simulink model "DeathOrGlory"  (R2017b)
settings: Solver=ode3  StartTime=0.0  StopTime=inf  FixedStep=0.0005  RelTol=1e-3
values from neighbouring files (symbols this model uses):
  fs = 1000    [Acquisizione_segnale_per_SVM_prova.m]    (also in training.m; warmup.m)
  interval = 192    [warmup.m]
  null_sum_finger = null_base_finger(:,1)+null_base_finger(:,2)    [matrix_h_hand_config.m]
  null_sum_thumb = null_base_thumb(:,1)+null_base_thumb(:,2)    [matrix_h_hand_config.m]
  num_act = 30    [KinematicData.m]
  pseudo_inv_h_finger = pinv(h_finger)    [matrix_h_hand_config.m]
  pseudo_inv_h_thumb = pinv(h_thumb)    [matrix_h_hand_config.m]
  pseudo_inv_h_wrist = pinv(h_wrist)    [matrix_h_hand_config.m]
  pseudo_inv_trasp_h_finger = pinv(transp(h_finger))    [matrix_h_hand_config.m]
  pseudo_inv_trasp_h_thumb = pinv(transp(h_thumb))    [matrix_h_hand_config.m]
  pseudo_inv_trasp_h_wrist = pinv(transp(h_wrist))    [matrix_h_hand_config.m]
  sM = mean(train(:,1:end-1))    [SVM_crossValidation.m]    (also in training.m; warmup.m = 0)
  sS = std(train(:,1:end-1))    [SVM_crossValidation.m]    (also in training.m; warmup.m = 0)
  Temg = 0.0005    [START_parametri_simulink.mat]    (also in matrix_h_hand_config.m)
  Ts = 0.05    [KinematicData.m]    (also in START_parametri_simulink.mat)
  w = 20    [Acquisizione_segnale_per_SVM_prova.m]    (also in warmup.m)
libraries: simulink x28, dspindex x15, dspfdesign x2, simulink_need_slupdate x2, dspmlti4 x1, dspstat3 x1, dspsrcs4 x1, simulink_extras x1
(part 1 of 2)
settings Model: Creator=UMBERTO  LastModifiedBy=Enrico
settings DataIOCC: LimitDataPoints=on  SaveFormat=Array
settings OptimizationCC: BlockReduction=off  BooleanDataType=off  LifeSpan=inf
settings DebuggingCC: SaveWithParameterizedLinksMsg=none  UnderspecifiedInitializationDetection=Classic  MergeDetectMultiDrivingBlocksExec=none  SignalResolutionControl=TryResolveAllWithWarning  SFUnexpectedBacktrackingDiag=warning  SFNoUnconditionalDefaultTransitionDiag=warning  SFExecutionAtInitializationDiag=none
settings HardwareCC: ProdBitPerPointer=32  ProdBitPerSizeT=32  ProdBitPerPtrDiffT=32  ProdLargestAtomicFloat=None  ProdIntDivRoundTo=Undefined  ProdEndianess=Unspecified  ProdWordSize=32  ProdHWDeviceType=32-bit Generic  TargetBitPerPointer=64  TargetBitPerSizeT=64  TargetBitPerPtrDiffT=64  TargetLongLongMode=on  TargetIntDivRoundTo=Zero  TargetEndianess=LittleEndian  TargetWordSize=64  TargetHWDeviceType=MATLAB Host  ProdEqTarget=off
settings ModelReferenceCC: UpdateModelReferenceTargets=Force  PropagateSignalLabelsOutOfModel=off
settings CodeAppCC: StateflowObjectComments=on
settings GRTTargetCC: TargetLangStandard=C89/C90 (ANSI)  GeneratePreprocessorConditionals=Disable all
settings ConfigComp: CovMetricSettings=dw  CovHtmlReporting=on  CovSaveCumulativeToWorkspaceVar=on  CovSaveSingleToWorkspaceVar=on  CovExternalEMLEnable=off  CovSFcnEnable=off

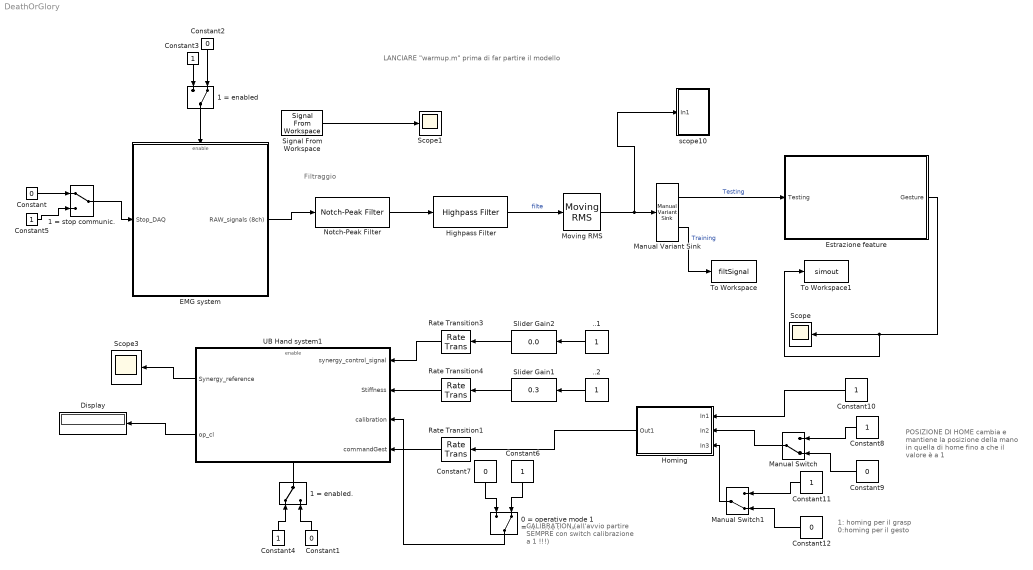
== system DeathOrGlory ==
  note: Filtraggio
  note: LANCIARE "warmup.m"
      | prima di far partire il modello
  note: CALIBRATION
      | (all'avvio partire SEMPRE con
      | switch calibrazione a 1 !!!)
  note: POSIZIONE DI HOME
      | cambia e mantiene la posizione della mano in quella di home fino a che il valore è a 1
  note: 1: homing per il grasp
      | 0:homing per il gesto
  ..1 : Constant  SampleTime=t
  ..2 : Constant  SampleTime=t
  0 = operative mode 1 = calibration mode : ManualSwitch  CurrentSetting=0
  1 = enabled : ManualSwitch  CurrentSetting=0  SampleTime=Temg
  1 = enabled. : ManualSwitch  SampleTime=t
  1 = stop communic. : ManualSwitch  SampleTime=Temg
  Constant : Constant  Value=0  SampleTime=Temg
  Constant1 : Constant  Value=0  SampleTime=t
  Constant{6,8,10..11} (4 alike) : Constant
  Constant12 : Constant  Value=0
  Constant2 : Constant  Value=0  SampleTime=Temg
  Constant3 : Constant  SampleTime=Temg
  Constant4 : Constant  SampleTime=t
  Constant5 : Constant  SampleTime=Temg
  Constant7 : Constant  Value=0
  Constant9 : Constant  Value=0
  Display : Display
  EMG system : Subsystem
  Estrazione feature : Subsystem
  Highpass Filter : dspfdesign/Highpass Filter  FilterType=FIR  DesignForMinimumOrder=on  FilterOrder=50  StopbandFrequency=w-5  PassbandFrequency=w  StopbandAttenuation=80  PassbandRipple=0.1  InheritSampleRate=off  SampleRate=fs  SimulateUsing=Interpreted execution  roundingMode=Floor  coeffsDataTypeStr=fixdt(1,16)
      settings: SourceProductName=DSP System Toolbox
  Homing : Subsystem
  Manual Variant Sink : simulink/Signal Routing/Manual Variant Sink  NumChoices=2  OverrideUsingVariant=V_1
      settings: SourceProductName=Simulink
  Manual Switch : ManualSwitch  CurrentSetting=0
  Manual Switch1 : ManualSwitch  CurrentSetting=0
  Moving RMS : dspstat3/Moving RMS  Method=Sliding window  SpecifyWindowLength=on  WindowLength=ws  ForgettingFactor=0.9  SimulateUsing=Code generation
      settings: SourceProductName=DSP System Toolbox  SourceProductBaseCode=DS
  Notch-Peak Filter : dspfdesign/Notch-Peak Filter  Specification=Quality factor and center frequency  Bandwidth=fs/2  QualityFactor=Q  CenterFrequency=notch  BandwidthCoefficient=0.72654  CenterFrequencyCoefficient=0  Output=Notch  InheritSampleRate=off  SampleRate=fs  SimulateUsing=Code generation
      settings: SourceProductName=DSP System Toolbox  SourceProductBaseCode=DS
  Rate Transition1 : RateTransition  OutPortSampleTime=Ts
  Rate Transition3 : RateTransition  OutPortSampleTime=Ts
  Rate Transition4 : RateTransition  OutPortSampleTime=Ts
  Scope : Scope
  Scope1 : Scope
  Scope3 : Scope
  Signal From Workspace : dspsrcs4/Signal From Workspace  X=cue_signal  Ts=1  nsamps=1  OutputAfterFinalValue=Cyclic repetition  ignoreOrWarnInputAndFrameLengths=off  OutputFrames=off
  Slider Gain1 : simulink/Math Operations/Slider Gain  gain=0.3  low=0  high=1
  Slider Gain2 : simulink/Math Operations/Slider Gain  gain=0.0  low=0  high=1
  To Workspace : ToWorkspace  VariableName=filtSignal  SampleTime=-1
      settings: Save2DSignal=2-D array (concatenate along first dimension)
  To Workspace1 : ToWorkspace  VariableName=simout  SampleTime=-1
      settings: Save2DSignal=2-D array (concatenate along first dimension)
  UB Hand system1 : Subsystem
  scope10 : Subsystem
  wires:
  Constant3/1 -> 1 = enabled/1
  Constant2/1 -> 1 = enabled/2
  1 = enabled/1 -> EMG system/Enable
  Constant5/1 -> 1 = stop communic./2
  Constant/1 -> 1 = stop communic./1
  1 = stop communic./1 -> EMG system/1(Stop_DAQ)
  Manual Variant Sink/2 -> To Workspace/1  "Training"
  Moving RMS/1 -> Manual Variant Sink/1, scope10/1(In1)
  Notch-Peak Filter/1 -> Highpass Filter/1
  Highpass Filter/1 -> Moving RMS/1  "filte"
  Constant4/1 -> 1 = enabled./1
  Slider Gain2/1 -> Rate Transition3/1
  ..1/1 -> Slider Gain2/1
  ..2/1 -> Slider Gain1/1
  Slider Gain1/1 -> Rate Transition4/1
  Constant6/1 -> 0 = operative mode 1 = calibration mode/2
  UB Hand system1/1(Synergy_reference) -> Scope3/1
  Constant1/1 -> 1 = enabled./2
  Rate Transition3/1 -> UB Hand system1/1(synergy_control_signal)
  Constant7/1 -> 0 = operative mode 1 = calibration mode/1
  Rate Transition4/1 -> UB Hand system1/2(Stiffness)
  UB Hand system1/2("op_cl ") -> Display/1
  0 = operative mode 1 = calibration mode/1 -> UB Hand system1/3(calibration)
  1 = enabled./1 -> UB Hand system1/Enable
  Rate Transition1/1 -> UB Hand system1/4(commandGest)
  Manual Variant Sink/1 -> Estrazione feature/1(Testing)  "Testing"
  Estrazione feature/1(Gesture) -> To Workspace1/1, Scope/1
  Constant8/1 -> Manual Switch/1
  Constant9/1 -> Manual Switch/2
  Manual Switch/1 -> Homing/2(In2)
  Manual Switch1/1 -> Homing/3(In3)
  Constant12/1 -> Manual Switch1/2
  Constant11/1 -> Manual Switch1/1
  Homing/1(Out1) -> Rate Transition1/1
  Constant10/1 -> Homing/1(In1)
  Signal From Workspace/1 -> Scope1/1
  EMG system/1(RAW_signals (8ch)) -> Notch-Peak Filter/1

== system DeathOrGlory/EMG system ==
  Stop_DAQ : Inport
  Enable : EnablePort
  MATLAB Function : MATLAB Function  TreatAsAtomicUnit=on
  Mux : Mux  Inputs=8
  RAW_signals (8ch) : Outport
  wires:
  Stop_DAQ/1 -> MATLAB Function/1(u)
  MATLAB Function/4(ch4) -> Mux/4
  MATLAB Function/3(ch3) -> Mux/3
  MATLAB Function/5(ch5) -> Mux/5
  MATLAB Function/6(ch6) -> Mux/6
  MATLAB Function/2(ch2) -> Mux/2
  MATLAB Function/1(ch1) -> Mux/1
  MATLAB Function/7(ch7) -> Mux/7
  MATLAB Function/8(ch8) -> Mux/8
  Mux/1 -> RAW_signals (8ch)/1

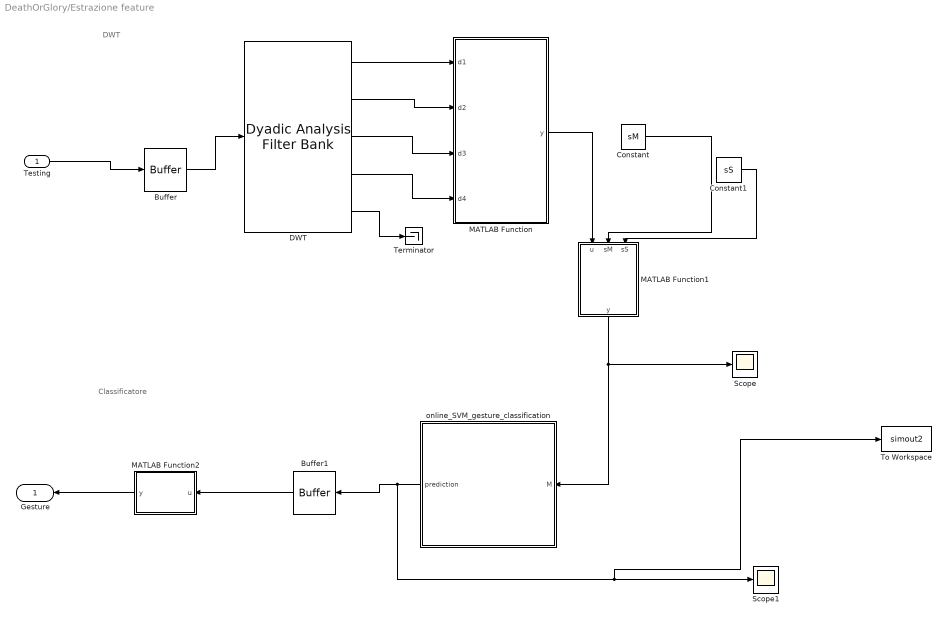
== system DeathOrGlory/Estrazione feature ==
  note: Classificatore
  note: DWT
  Testing : Inport
  Buffer : Buffer  N=interval  V=over  OutputFrames=off
  Buffer1 : Buffer  N=35  V=34
  Constant : Constant  Value=sM
  Constant1 : Constant  Value=sS
  DWT : dspmlti4/Dyadic Analysis Filter Bank  Wname=Daubechies  OrdRec_ordDec=[1 / 1]  Order=3  LPF="[0.0352   -0.0854   -0.1350   0.4599   0.8069   0.3327]"  HPF="[-0.3327    0.8069   -0.4599   -0.1350    0.0854    0.0352]"  NumLevels=level_dec  tree=Asymmetric  Output=Multiple ports  OutputFrames=off
      settings: SourceProductName=DSP System Toolbox  SourceProductBaseCode=DS
  MATLAB Function : MATLAB Function  TreatAsAtomicUnit=on
  MATLAB Function1 : MATLAB Function  TreatAsAtomicUnit=on
  MATLAB Function2 : MATLAB Function  TreatAsAtomicUnit=on
  Scope : Scope
  Scope1 : Scope
  Terminator : Terminator
  To Workspace : ToWorkspace  VariableName=simout2  SampleTime=-1
      settings: Save2DSignal=2-D array (concatenate along first dimension)
  online_SVM_gesture_classification : MATLAB Function  TreatAsAtomicUnit=on
  Gesture : Outport
  wires:
  DWT/5 -> Terminator/1
  DWT/3 -> MATLAB Function/3(d3)
  MATLAB Function/1(y) -> MATLAB Function1/1(u)
  DWT/1 -> MATLAB Function/1(d1)
  DWT/4 -> MATLAB Function/4(d4)
  DWT/2 -> MATLAB Function/2(d2)
  Buffer/1 -> DWT/1
  Testing/1 -> Buffer/1
  Buffer1/1 -> MATLAB Function2/1(u)
  online_SVM_gesture_classification/1(prediction) -> To Workspace/1, Scope1/1, Buffer1/1
  MATLAB Function1/1(y) -> Scope/1, online_SVM_gesture_classification/1(M)
  MATLAB Function2/1(y) -> Gesture/1
  Constant/1 -> MATLAB Function1/2(sM)
  Constant1/1 -> MATLAB Function1/3(sS)

== system DeathOrGlory/Homing ==
  In1 : Inport
  In2 : Inport  Port=2
  In3 : Inport  Port=3
  Constant : Constant  Value=8
  Constant1 : Constant
  Delay : Delay
  MATLAB Function : MATLAB Function  TreatAsAtomicUnit=on
  Scope : Scope
  Switch : Switch  Criteria=u2 ~= 0
  Switch1 : Switch  Criteria=u2 ~= 0
  Out1 : Outport
  wires:
  Delay/1 -> MATLAB Function/2(out)
  MATLAB Function/1(y) -> Switch/3
  In2/1 -> Switch/2
  Switch/1 -> Out1/1, Scope/1, Delay/1
  Constant1/1 -> Switch1/1
  Constant/1 -> Switch1/3
  In3/1 -> Switch1/2
  Switch1/1 -> Switch/1
  In1/1 -> MATLAB Function/1(u)

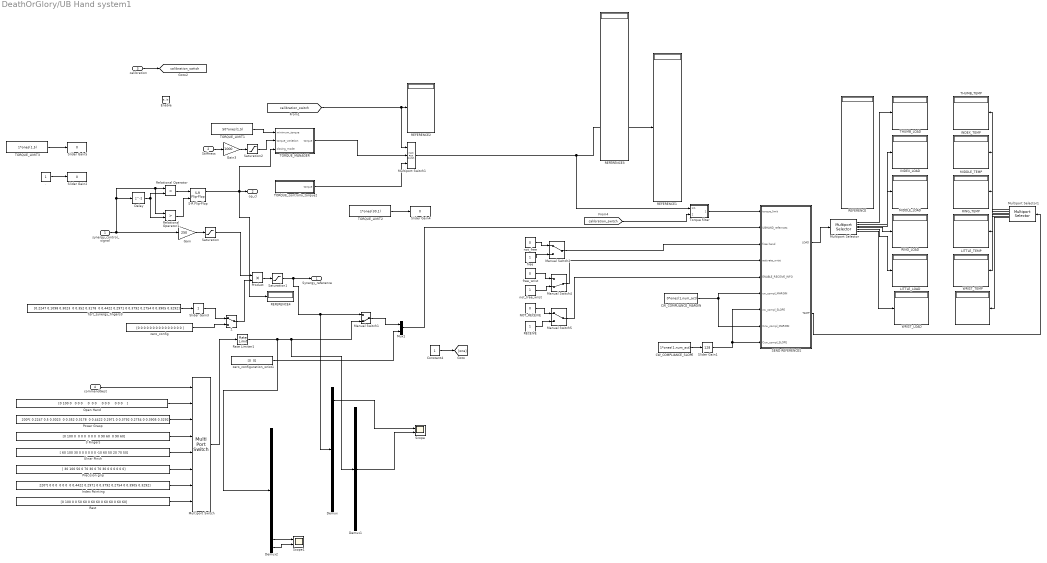
== system DeathOrGlory/UB Hand system1 ==
  synergy_control_signal : Inport
  Stiffness : Inport  Port=2
  calibration : Inport  Port=3
  commandGest : Inport  Port=4
  Enable : EnablePort
  . : Constant  SampleTime=t
  3 Fingers : Constant  Value="[0 100 0  0 0 0  0 0 0  0 90 60  0 90 60]"  SampleTime=t
  :1 : ManualSwitch  SampleTime=t
  CW_COMPLIANCE_MARGIN : Constant  Value=0*ones(1,num_act)
  CW_COMPLIANCE_SLOPE : Constant  Value=1*ones(1,num_act)
  Constant4 : Constant  SampleTime=t
  Delay : Delay  DelayLength=1  InitialCondition=0
  Demux : Demux  Outputs=15
  Demux1 : Demux  Outputs=15
  Demux2 : Demux  Outputs=15
  Gain : Gain  Gain=250
  Gain3 : Gain  Gain=1000
  INDEX_LOAD : Display
  INDEX_TEMP : Display
  Index Pointing : Constant  Value="220*[ 0 0 0  0 0 0  0 0.4422 0.2971 0 0.3792 0.2754 0 0.3905 0.3292]"  SampleTime=t
  LITTLE_LOAD : Display
  LITTLE_TEMP : Display
  MIDDLE_LOAD : Display
  MIDDLE_TEMP : Display
  Manual Switch1 : ManualSwitch  CurrentSetting=0
  Manual Switch2 : ManualSwitch  Description=SEND  SampleTime=t
      settings: AttributesFormatString=SEND
  Manual Switch4 : ManualSwitch  Description=SEND  CurrentSetting=0  SampleTime=t
      settings: AttributesFormatString=SEND
  Manual Switch5 : ManualSwitch  Description=SEND  SampleTime=t
      settings: AttributesFormatString=SEND
  Multiport Selector : dspindex/Multiport Selector  rowsOrCols=Rows  idxCellArray={ [1:5],[6:10],[11:15],[16:20],[21:25],[26:29]}  idxErrMode=Clip Index
  Multiport Selector1 : dspindex/Multiport Selector  rowsOrCols=Rows  idxCellArray={ [1:5],[6:10],[11:15],[16:20],[21:25],[26:29]}  idxErrMode=Clip Index
  Multiport Switch : MultiPortSwitch  DataPortOrder=Specify indices  Inputs=6  DataPortIndices={1,2,3,4,5,6,8}
  Multiport Switch1 : MultiPortSwitch  DataPortOrder=Zero-based contiguous  Inputs=2  DiagnosticForDefault=None
  Mux1 : Mux  Inputs=2
  NOT_RECEIVE : Constant  Value=0  SampleTime=t
  Open Hand : Constant  Value="[0 100 0   0 0 0     0  0 0     0 0 0     0 0 0    ]"  SampleTime=t
  Power Grasp : Constant  Value="200*[ 0.2247 0.5 0.3023  0 0.352 0.3178  0 0.4422 0.2971 0 0.3792 0.2754 0 0.3905 0.3292]"  SampleTime=t
  Precision grip : Constant  Value=[ 30 100 50 0 70 30 0 70 30 0 0 0 0 0 0]  SampleTime=t
  Product : Product  SampleTime=t
  RECEIVE : Constant  SampleTime=t
  REFERENCE{,1..4} (5 alike) : Display
  RING_LOAD : Display
  RING_TEMP : Display
  Rate Limiter1 : RateLimiter  RisingSlewLimit=80  FallingSlewLimit=-80  SampleTimeMode=inherited
  Relational Operator : RelationalOperator  Operator=<  OutDataTypeStr=boolean  RndMeth=Nearest
  Relational Operator1 : RelationalOperator  Operator=>  OutDataTypeStr=boolean  RndMeth=Nearest
  Rest : Constant  Value=[0 100 0 0 50 60 0 60 60 0 60 60 0 60 60]  SampleTime=t
  S-R Flip-Flop : simulink_extras/Flip Flops/S-R Flip-Flop  initial_condition=0
  SEND REFERENCES : Subsystem
  Saturation : Saturate  UpperLimit=250  LowerLimit=0
  Saturation1 : Saturate  UpperLimit=250  LowerLimit=0
  Saturation2 : Saturate  UpperLimit=1000  LowerLimit=0
  Scope : Scope  NumInputPorts=2
  Scope1 : Scope  NumInputPorts=2
  Slider Gain1 : simulink/Math Operations/Slider Gain  gain=128  low=0  high=128
  Slider Gain2 : simulink/Math Operations/Slider Gain  gain=0  low=0  high=1000
  Slider Gain3 : simulink/Math Operations/Slider Gain  gain=1  low=0  high=250
  Slider Gain4 : simulink/Math Operations/Slider Gain  gain=0  low=0  high=1000
  Slider Gain5 : simulink/Math Operations/Slider Gain  gain=0  low=0  high=1000
  THUMB_LOAD : Display
  THUMB_TEMP : Display
  TORQUE_LIMIT1 : Constant  Value=50*ones(1,5)  SampleTime=t
  TORQUE_LIMIT2 : Constant  Value=1*ones(30,1)  SampleTime=t
  TORQUE_LIMIT3 : Constant  Value=1*ones(1,5)  SampleTime=t
  TORQUE_MANAGER : Subsystem
  TORQUE_controllo_torque2 : Subsystem
  Torque filter : Subsystem
  Ulnar Pinch : Constant  Value=[ 60 100 30 0 0 0 0 0 0 -10 60 50 20 70 50]  SampleTime=t
  WRIST_LOAD : Display
  WRIST_TEMP : Display
  fisrt_synergy_fingers3 : Constant  Value="[0.2247 0.1098 0.3023  0 0.352 0.3178  0 0.4422 0.2971 0 0.3792 0.2754 0 0.3905 0.3292]'"  SampleTime=t
  free : Constant  SampleTime=t
  free_wrist : Constant  Value=0  SampleTime=t
  not_free : Constant  Value=0  SampleTime=t
  not_free_wrist : Constant  SampleTime=t
  zero_config : Constant  Value="[0 0 0   0 0 0     0  0 0     0 0 0     0 0 0    ]"  SampleTime=t
  zero_configuration_wrist1 : Constant  Value="[0  0]"  SampleTime=t
  Synergy_reference : Outport
  "op_cl " : Outport  Port=2
  tag scope: calibration_switch=global
  wires:
  Constant4/1 -> [one]
  not_free/1 -> Manual Switch2/1
  free/1 -> Manual Switch2/2
  Manual Switch2/1 -> SEND REFERENCES/3(free hand)
  free_wrist/1 -> Manual Switch4/1
  Manual Switch4/1 -> SEND REFERENCES/4(activate_wrist)
  NOT_RECEIVE/1 -> Manual Switch5/1
  RECEIVE/1 -> Manual Switch5/2
  Manual Switch5/1 -> SEND REFERENCES/5(ENABLE_RECEIVE_INFO)
  not_free_wrist/1 -> Manual Switch4/2
  zero_configuration_wrist1/1 -> Mux1/2
  Gain/1 -> Saturation/1
  SEND REFERENCES/2(TEMP) -> Multiport Selector1/1
  Multiport Selector/1 -> THUMB_LOAD/1
  Multiport Selector/2 -> INDEX_LOAD/1
  Multiport Selector/3 -> MIDDLE_LOAD/1
  Multiport Selector/4 -> RING_LOAD/1
  Multiport Selector/5 -> LITTLE_LOAD/1
  Multiport Selector/6 -> WRIST_LOAD/1
  Multiport Selector1/1 -> THUMB_TEMP/1
  Multiport Selector1/2 -> INDEX_TEMP/1
  Multiport Selector1/3 -> MIDDLE_TEMP/1
  Multiport Selector1/4 -> RING_TEMP/1
  Multiport Selector1/5 -> LITTLE_TEMP/1
  Multiport Selector1/6 -> WRIST_TEMP/1
  SEND REFERENCES/1(LOAD) -> Multiport Selector/1
  Saturation/1 -> Product/1
  CW_COMPLIANCE_SLOPE/1 -> Slider Gain1/1
  TORQUE_LIMIT1/1 -> TORQUE_MANAGER/1(minimum_torque)
  [calibration_switch] -> Multiport Switch1/1, REFERENCE2/1
  Product/1 -> Saturation1/1
  Saturation1/1 -> Demux/1, Manual Switch1/1, Synergy_reference/1
  TORQUE_controllo_torque2/1(torque) -> Multiport Switch1/3
  zero_config/1 -> :1/2
  :1/1 -> Product/2
  fisrt_synergy_fingers3/1 -> Slider Gain3/1
  TORQUE_LIMIT2/1 -> Slider Gain4/1
  TORQUE_LIMIT3/1 -> Slider Gain5/1
  ./1 -> Slider Gain2/1
  Saturation2/1 -> TORQUE_MANAGER/2(torque_variation)
  Mux1/1 -> SEND REFERENCES/2(UBHAND_refernces)
  CW_COMPLIANCE_MARGIN/1 -> SEND REFERENCES/6(cw_compl_MARGIN), SEND REFERENCES/8(Ccw_compl_MARGIN)
  Slider Gain1/1 -> SEND REFERENCES/7("cw_compl_SLOPE "), SEND REFERENCES/9(Ccw_compl_SLOPE)
  Torque filter/1(Out1) -> SEND REFERENCES/1(torque_limit)
  [calibration_switch] -> Torque filter/2("reset ")
  calibration/1 -> [calibration_switch]
  Multiport Switch1/1 -> Torque filter/1(In1), REFERENCE1/1
  TORQUE_MANAGER/1(torque) -> Multiport Switch1/2
  Gain3/1 -> Saturation2/1
  Stiffness/1 -> Gain3/1
  Slider Gain3/1 -> :1/1
  Delay/1 -> Relational Operator1/2, Relational Operator/2
  S-R Flip-Flop/1 -> TORQUE_MANAGER/3(closing_mode), "op_cl "/1, REFERENCE4/1
  Relational Operator/1 -> S-R Flip-Flop/1
  synergy_control_signal/1 -> Relational Operator1/1, Relational Operator/1, Delay/1, Gain/1
  Relational Operator1/1 -> S-R Flip-Flop/2
  Multiport Switch/1 -> Rate Limiter1/1
  Manual Switch1/1 -> Mux1/1
  Demux/2 -> Scope/1
  Demux1/8 -> Scope/2
  Open Hand/1 -> Multiport Switch/2
  Power Grasp/1 -> Multiport Switch/3
  3 Fingers/1 -> Multiport Switch/4
  Ulnar Pinch/1 -> Multiport Switch/5
  Precision grip/1 -> Multiport Switch/6
  Index Pointing/1 -> Multiport Switch/7
  Rest/1 -> Multiport Switch/8
  commandGest/1 -> Multiport Switch/1
  Rate Limiter1/1 -> Demux2/1, Demux1/1, Manual Switch1/2
  Demux2/14 -> Scope1/1
  Demux2/15 -> Scope1/2

== system DeathOrGlory/scope10 ==
  In1 : Inport
  Demux : Demux  Outputs=8
  Scope : Scope  NumInputPorts=8
  wires:
  In1/1 -> Demux/1
  Demux/7 -> Scope/7
  Demux/4 -> Scope/4
  Demux/5 -> Scope/5
  Demux/8 -> Scope/8
  Demux/1 -> Scope/1
  Demux/2 -> Scope/2
  Demux/6 -> Scope/6
  Demux/3 -> Scope/3

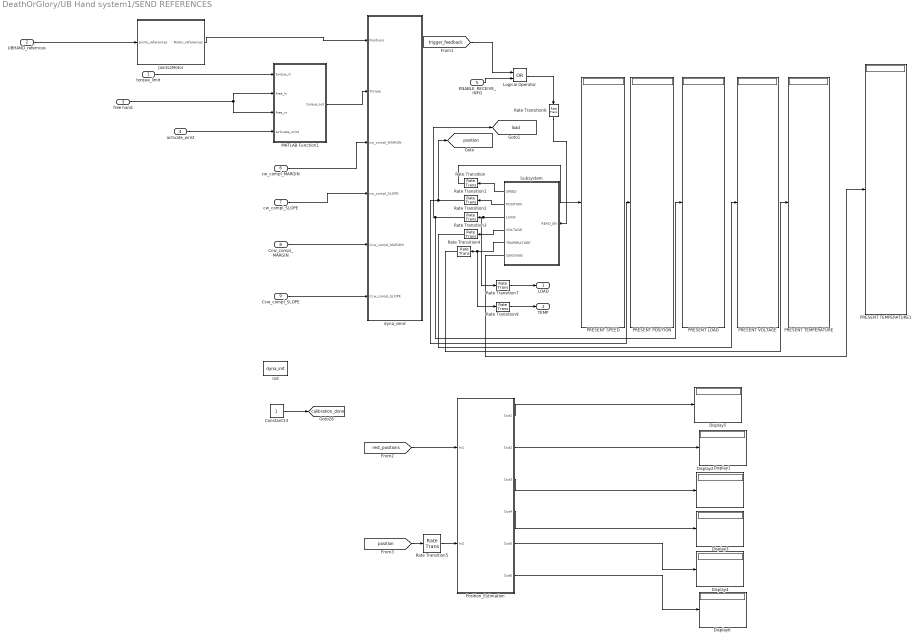
== system DeathOrGlory/UB Hand system1/SEND REFERENCES ==
  torque_limit : Inport
  UBHAND_refernces : Inport  Port=2
  free hand : Inport  Port=3
  activate_wrist : Inport  Port=4
  ENABLE_RECEIVE_INFO : Inport  Port=5
  cw_compl_MARGIN : Inport  Port=6
  "cw_compl_SLOPE " : Inport  Port=7
  Ccw_compl_MARGIN : Inport  Port=8
  Ccw_compl_SLOPE : Inport  Port=9
  Constant33 : Constant  SampleTime=Ts
  Display{1..6} (6 alike) : Display
  Init : M-S-Function  FunctionName=dyna_init  Parameters=5 1
  Joints2Motor : Subsystem
  Logical Operator : Logic  Operator=OR  AllPortsSameDT=off  OutDataTypeStr=boolean
  MATLAB Function1 : MATLAB Function  TreatAsAtomicUnit=on
  PRESENT LOAD : Display
  PRESENT POSITION : Display
  PRESENT SPEED : Display
  PRESENT TEMPERATURE : Display
  PRESENT TEMPERATURE1 : Display
  PRESENT VOLTAGE : Display
  Position_Estimation : Subsystem
  Rate Transition{,1..4,6..7,9} (8 alike) : RateTransition
  Rate Transition5 : RateTransition  OutPortSampleTime=Ts
  Subsystem : Subsystem  SystemSampleTime=0.1
  dyna_send : Subsystem
  LOAD : Outport
  TEMP : Outport  Port=2
  tag scope: calibration_done=global, load=global, position=global
  wires:
  torque_limit/1 -> MATLAB Function1/1(torque_in)
  Joints2Motor/1(Motor_references) -> dyna_send/1(Positions)
  ENABLE_RECEIVE_INFO/1 -> Logical Operator/2
  Logical Operator/1 -> Rate Transition6/1
  [trigger_feedback] -> Logical Operator/1
  activate_wrist/1 -> MATLAB Function1/4(activate_wrist)
  MATLAB Function1/1(torque_out) -> dyna_send/2(Torque)
  UBHAND_refernces/1 -> Joints2Motor/1(Joints_references)
  free hand/1 -> MATLAB Function1/3(free_rx), MATLAB Function1/2(free_lx)
  Constant33/1 -> [calibration_done]
  Subsystem/1(SPEED) -> Rate Transition/1
  Subsystem/2(POSITION) -> Rate Transition1/1
  Subsystem/3(LOAD) -> Rate Transition7/1, Rate Transition2/1
  Subsystem/4(VOLTAGE) -> Rate Transition3/1
  Subsystem/5(TEMPERATURE) -> Rate Transition4/1, Rate Transition9/1
  cw_compl_MARGIN/1 -> dyna_send/3(cw_compl_MARGIN)
  "cw_compl_SLOPE "/1 -> dyna_send/4(cw_compl_SLOPE)
  Ccw_compl_MARGIN/1 -> dyna_send/5(Ccw_compl_MARGIN)
  Ccw_compl_SLOPE/1 -> dyna_send/6(Ccw_compl_SLOPE)
  Position_Estimation/1(Out1) -> Display5/1
  Position_Estimation/2(Out2) -> Display1/1
  Position_Estimation/3(Out3) -> Display2/1
  Position_Estimation/4(Out4) -> Display3/1
  Position_Estimation/5(Out5) -> Display4/1
  Position_Estimation/6(Out6) -> Display6/1
  [rest_positions] -> Position_Estimation/1(In1)
  [position] -> Rate Transition5/1
  Rate Transition/1 -> PRESENT SPEED/1
  Rate Transition1/1 -> [position], PRESENT POSITION/1
  Rate Transition3/1 -> PRESENT VOLTAGE/1
  Rate Transition4/1 -> PRESENT TEMPERATURE/1
  Rate Transition5/1 -> Position_Estimation/2(In2)
  Rate Transition6/1 -> Subsystem/1(READ_EN)
  Rate Transition9/1 -> TEMP/1
  Rate Transition7/1 -> LOAD/1
  Rate Transition2/1 -> [load], PRESENT LOAD/1
  Subsystem/6(ISMOVING) -> PRESENT TEMPERATURE1/1

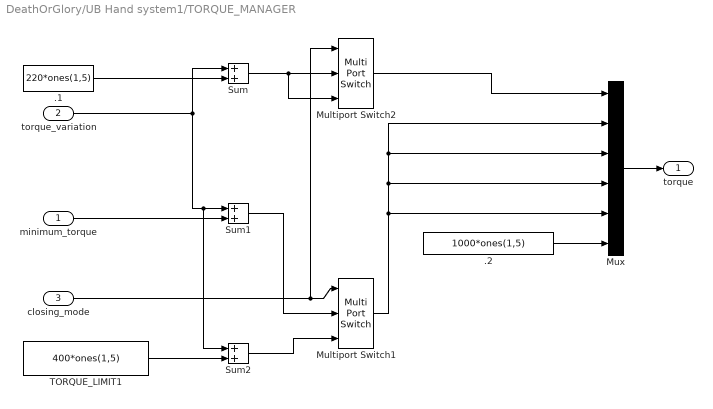
== system DeathOrGlory/UB Hand system1/TORQUE_MANAGER ==
  minimum_torque : Inport
  torque_variation : Inport  Port=2
  closing_mode : Inport  Port=3
  .1 : Constant  Value=220*ones(1,5)  SampleTime=t
  .2 : Constant  Value=1000*ones(1,5)  SampleTime=t
  Multiport Switch1 : MultiPortSwitch  DataPortOrder=Zero-based contiguous  Inputs=2  DiagnosticForDefault=None
  Multiport Switch2 : MultiPortSwitch  DataPortOrder=Zero-based contiguous  Inputs=2  DiagnosticForDefault=None
  Mux : Mux  Inputs=6
  Sum : Sum
  Sum1 : Sum
  Sum2 : Sum
  TORQUE_LIMIT1 : Constant  Value=400*ones(1,5)  SampleTime=t
  torque : Outport
  wires:
  Mux/1 -> torque/1
  .1/1 -> Sum/2
  minimum_torque/1 -> Sum1/2
  torque_variation/1 -> Sum2/1, Sum1/1, Sum/1
  .2/1 -> Mux/6
  closing_mode/1 -> Multiport Switch2/1, Multiport Switch1/1
  Sum1/1 -> Multiport Switch1/2
  Multiport Switch1/1 -> Mux/5, Mux/4, Mux/3, Mux/2
  Sum/1 -> Multiport Switch2/3, Multiport Switch2/2
  Multiport Switch2/1 -> Mux/1
  TORQUE_LIMIT1/1 -> Sum2/2
  Sum2/1 -> Multiport Switch1/3

== system DeathOrGlory/UB Hand system1/TORQUE_controllo_torque2 ==
  Display{1..6} (6 alike) : Display
  Mux : Mux  Inputs=6
  Ring_proximal_back_forward2 : Constant  SampleTime=-1
  Subsystem1 : Subsystem
  torque : Outport
  wires:
  Subsystem1/2(tau_index) -> Display1/1, Mux/2
  Mux/1 -> torque/1
  Subsystem1/6(tau_wrist) -> Display6/1, Mux/6
  Subsystem1/5(tau_little) -> Display5/1, Mux/5
  Subsystem1/4(tau_ring) -> Display4/1, Mux/4
  Subsystem1/3(tau_middle) -> Display3/1, Mux/3
  Subsystem1/1(tau_thumb) -> Display2/1, Mux/1
  Ring_proximal_back_forward2/1 -> [one]

== system DeathOrGlory/UB Hand system1/Torque filter ==
  In1 : Inport
  "reset " : Inport  Port=2
  Detect Increase : simulink/Logic and Bit Operations/Detect Increase  vinit=0.0  InputProcessing=Inherited  OutDataTypeStr=boolean
  Fc2 : Constant  Value=0.1  SampleTime=-1
  First Order Filtering1 : Subsystem
  Fs2 : Constant  Value=1/Ts  SampleTime=-1
  Out1 : Outport
  wires:
  Fc2/1 -> First Order Filtering1/2(Fc)
  Fs2/1 -> First Order Filtering1/3(Fs)
  In1/1 -> First Order Filtering1/1(X)
  First Order Filtering1/1(y) -> Out1/1
  "reset "/1 -> Detect Increase/1
  Detect Increase/1 -> First Order Filtering1/4(reset)

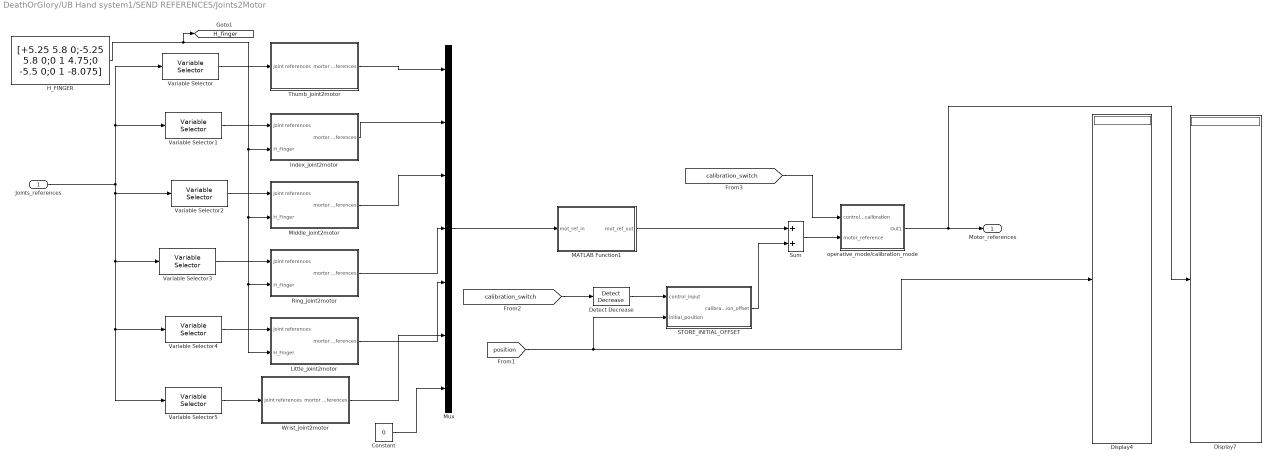
== system DeathOrGlory/UB Hand system1/SEND REFERENCES/Joints2Motor ==
  Joints_references : Inport
  Constant : Constant  Value=0  SampleTime=t
  Detect Decrease : simulink/Logic and Bit Operations/Detect Decrease  vinit=0.0  InputProcessing=Inherited  OutDataTypeStr=boolean
  Display4 : Display
  Display7 : Display
  H_FINGER : Constant  Value=[+5.25 5.8 0;-5.25 5.8 0;0 1 4.75;0 -5.5 0;0 1 -8.075]  VectorParams1D=off  SampleTime=t
  Index_joint2motor : Subsystem
  Little_joint2motor : Subsystem
  MATLAB Function1 : MATLAB Function  TreatAsAtomicUnit=on
  Middle_joint2motor : Subsystem
  Mux : Mux  Inputs=7
  Ring_joint2motor : Subsystem
  STORE_INITIAL_OFFSET : Subsystem
  Sum : Sum
  Thumb_joint2motor : Subsystem
  Variable Selector : dspindex/Variable Selector  NumInputs=1  rowsOrCols=Rows  IdxMode=Fixed  Elements=[1:3]  ZerOneIdxMode=One-based  errmode=Clip Index  FillMode=on  FillValues=0
  Variable Selector1 : dspindex/Variable Selector  NumInputs=1  rowsOrCols=Rows  IdxMode=Fixed  Elements=[4:6]  ZerOneIdxMode=One-based  errmode=Clip Index  FillMode=on  FillValues=0
  Variable Selector2 : dspindex/Variable Selector  NumInputs=1  rowsOrCols=Rows  IdxMode=Fixed  Elements=[7:9]  ZerOneIdxMode=One-based  errmode=Clip Index  FillMode=on  FillValues=0
  Variable Selector3 : dspindex/Variable Selector  NumInputs=1  rowsOrCols=Rows  IdxMode=Fixed  Elements=[10:12]  ZerOneIdxMode=One-based  errmode=Clip Index  FillMode=on  FillValues=0
  Variable Selector4 : dspindex/Variable Selector  NumInputs=1  rowsOrCols=Rows  IdxMode=Fixed  Elements=[13:15]  ZerOneIdxMode=One-based  errmode=Clip Index  FillMode=on  FillValues=0
  Variable Selector5 : dspindex/Variable Selector  NumInputs=1  rowsOrCols=Rows  IdxMode=Fixed  Elements=[16:17]  ZerOneIdxMode=One-based  errmode=Clip Index  FillMode=on  FillValues=0
  Wrist_joint2motor : Subsystem
  operative_mode/calibration_mode : Subsystem
  Motor_references : Outport
  tag scope: H_finger=global
  wires:
  Wrist_joint2motor/1(mortor references) -> Mux/6
  Little_joint2motor/1(mortor references) -> Mux/5
  Ring_joint2motor/1(mortor references) -> Mux/4
  Middle_joint2motor/1(mortor references) -> Mux/3
  Index_joint2motor/1(mortor references) -> Mux/2
  Thumb_joint2motor/1(mortor references) -> Mux/1
  Mux/1 -> MATLAB Function1/1(mot_ref_in)
  Variable Selector5/1 -> Wrist_joint2motor/1(Joint references)
  Variable Selector4/1 -> Little_joint2motor/1(Joint references)
  Variable Selector3/1 -> Ring_joint2motor/1(Joint references)
  Variable Selector2/1 -> Middle_joint2motor/1(Joint references)
  Variable Selector1/1 -> Index_joint2motor/1(Joint references)
  Variable Selector/1 -> Thumb_joint2motor/1(Joint references)
  Constant/1 -> Mux/7
  H_FINGER/1 -> Index_joint2motor/2(H_Finger), Little_joint2motor/2(H_Finger), Ring_joint2motor/2(H_Finger), Middle_joint2motor/2(H_Finger), [H_finger]
  Joints_references/1 -> Variable Selector1/1, Variable Selector/1, Variable Selector2/1, Variable Selector3/1, Variable Selector4/1, Variable Selector5/1
  MATLAB Function1/1(mot_ref_out) -> Sum/1
  [calibration_switch] -> operative_mode/calibration_mode/1(control_calibration)
  STORE_INITIAL_OFFSET/1(calibration_offset) -> Sum/2
  operative_mode/calibration_mode/1(Out1) -> Motor_references/1, Display7/1
  Sum/1 -> operative_mode/calibration_mode/2(motor_reference)
  [position] -> Display4/1, STORE_INITIAL_OFFSET/2(initial_position)
  [calibration_switch] -> Detect Decrease/1
  Detect Decrease/1 -> STORE_INITIAL_OFFSET/1(control_input)

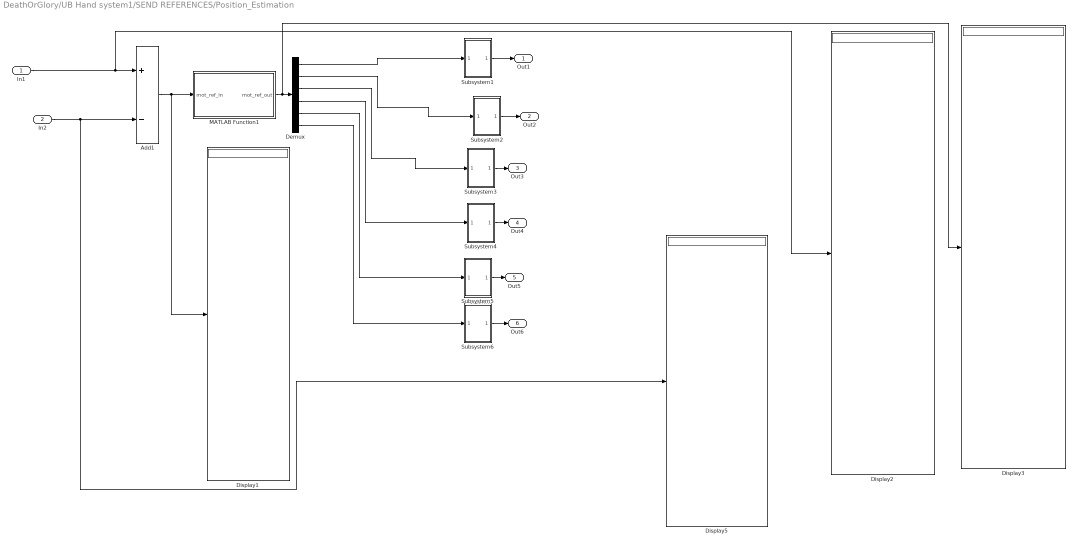
== system DeathOrGlory/UB Hand system1/SEND REFERENCES/Position_Estimation ==
  In1 : Inport
  In2 : Inport  Port=2
  Add1 : Sum  Inputs=+-
  Demux : Demux  Outputs=6
  Display{1..3,5} (4 alike) : Display
  MATLAB Function1 : MATLAB Function  TreatAsAtomicUnit=on
  Subsystem1 : Subsystem
  Subsystem2 : Subsystem
  Subsystem3 : Subsystem
  Subsystem4 : Subsystem
  Subsystem5 : Subsystem
  Subsystem6 : Subsystem
  Out1 : Outport
  Out2 : Outport  Port=2
  Out3 : Outport  Port=3
  Out4 : Outport  Port=4
  Out5 : Outport  Port=5
  Out6 : Outport  Port=6
  wires:
  Demux/1 -> Subsystem1/1(In1)
  Demux/2 -> Subsystem2/1(In1)
  Demux/3 -> Subsystem3/1(In1)
  Demux/4 -> Subsystem4/1(In1)
  Demux/5 -> Subsystem5/1(In1)
  Add1/1 -> Display1/1, MATLAB Function1/1(mot_ref_in)
  Demux/6 -> Subsystem6/1(In1)
  In1/1 -> Display2/1, Add1/1
  Subsystem1/1(Out1) -> Out1/1
  Subsystem2/1(Out1) -> Out2/1
  Subsystem3/1(Out1) -> Out3/1
  Subsystem4/1(Out1) -> Out4/1
  Subsystem5/1(Out1) -> Out5/1
  Subsystem6/1(Out1) -> Out6/1
  In2/1 -> Display5/1, Add1/2
  MATLAB Function1/1(mot_ref_out) -> Display3/1, Demux/1

== system DeathOrGlory/UB Hand system1/SEND REFERENCES/Subsystem ==
  READ_EN : Inport
  Triggered Subsystem : Subsystem  TreatAsAtomicUnit=on
  SPEED : Outport
  POSITION : Outport  Port=2
  LOAD : Outport  Port=3
  VOLTAGE : Outport  Port=4
  TEMPERATURE : Outport  Port=5
  ISMOVING : Outport  Port=6
  wires:
  Triggered Subsystem/2(Out3) -> POSITION/1
  Triggered Subsystem/3(Out4) -> LOAD/1
  READ_EN/1 -> Triggered Subsystem/Enable
  Triggered Subsystem/1(Out2) -> SPEED/1
  Triggered Subsystem/4(Out5) -> VOLTAGE/1
  Triggered Subsystem/5(Out6) -> TEMPERATURE/1
  Triggered Subsystem/6(IsMoving) -> ISMOVING/1

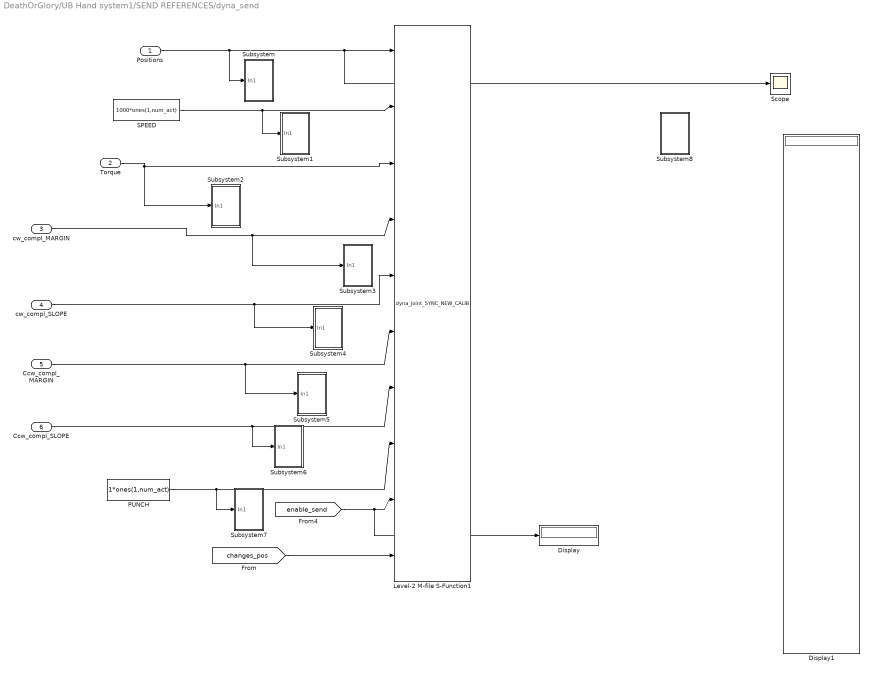
== system DeathOrGlory/UB Hand system1/SEND REFERENCES/dyna_send ==
  Positions : Inport
  Torque : Inport  Port=2
  cw_compl_MARGIN : Inport  Port=3
  cw_compl_SLOPE : Inport  Port=4
  Ccw_compl_MARGIN : Inport  Port=5
  Ccw_compl_SLOPE : Inport  Port=6
  Display : Display
  Display1 : Display
  Level-2 M-file S-Function1 : M-S-Function  FunctionName=dyna_joint_SYNC_NEW_CALIB  Parameters=[13 14 10 12 11 8 9 7 5 6 2 4 3 27 28 24 26 25 21 23 20 22 19 17 18 15 16 1 30 29]
  PUNCH : Constant  Value=1*ones(1,num_act)
  SPEED : Constant  Value=1000*ones(1,num_act)
  Scope : Scope
  Subsystem : Subsystem
  Subsystem1 : Subsystem
  Subsystem2 : Subsystem
  Subsystem3 : Subsystem
  Subsystem4 : Subsystem
  Subsystem5 : Subsystem
  Subsystem6 : Subsystem
  Subsystem7 : Subsystem
  Subsystem8 : Subsystem
  wires:
  cw_compl_MARGIN/1 -> Level-2 M-file S-Function1/4, Subsystem3/1(In1)
  Ccw_compl_MARGIN/1 -> Level-2 M-file S-Function1/6, Subsystem5/1(In1)
  PUNCH/1 -> Level-2 M-file S-Function1/8, Subsystem7/1(In1)
  Positions/1 -> Subsystem/1(In1), Level-2 M-file S-Function1/1, Scope/1
  [enable_send] -> Level-2 M-file S-Function1/9, Display/1
  [changes_pos] -> Level-2 M-file S-Function1/10
  Ccw_compl_SLOPE/1 -> Level-2 M-file S-Function1/7, Subsystem6/1(In1)
  cw_compl_SLOPE/1 -> Level-2 M-file S-Function1/5, Subsystem4/1(In1)
  SPEED/1 -> Level-2 M-file S-Function1/2, Subsystem1/1(In1)
  Torque/1 -> Subsystem2/1(In1), Level-2 M-file S-Function1/3

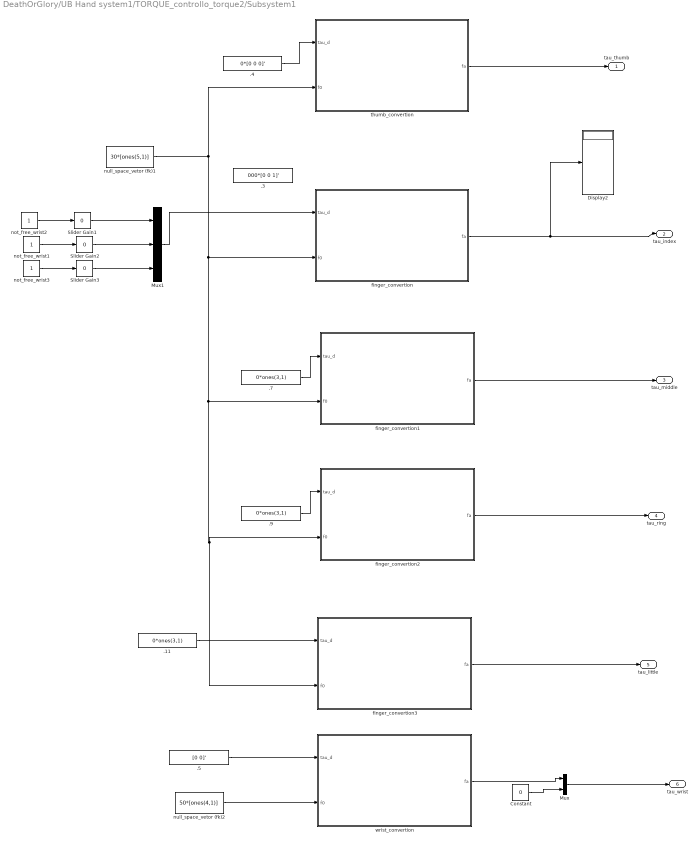
== system DeathOrGlory/UB Hand system1/TORQUE_controllo_torque2/Subsystem1 ==
  .11 : Constant  Value=0*ones(3,1)  VectorParams1D=off  SampleTime=-1
  .3 : Constant  Value=000*[0 0 1]'  VectorParams1D=off  SampleTime=-1
  .4 : Constant  Value=0*[0 0 0]'  VectorParams1D=off  SampleTime=-1
  .5 : Constant  Value=[0 0]'  VectorParams1D=off  SampleTime=-1
  .7 : Constant  Value=0*ones(3,1)  VectorParams1D=off  SampleTime=-1
  .9 : Constant  Value=0*ones(3,1)  VectorParams1D=off  SampleTime=-1
  Constant : Constant  Value=0
  Display2 : Display
  Mux : Mux  Inputs=2
  Mux1 : Mux  Inputs=3
  Slider Gain1 : simulink/Math Operations/Slider Gain  gain=0  low=0  high=11
  Slider Gain2 : simulink/Math Operations/Slider Gain  gain=0  low=-10000  high=10000
  Slider Gain3 : simulink/Math Operations/Slider Gain  gain=0  low=-10000  high=50000
  finger_convertion : Subsystem
  finger_convertion1 : Subsystem
  finger_convertion2 : Subsystem
  finger_convertion3 : Subsystem
  not_free_wrist1 : Constant  SampleTime=t
  not_free_wrist2 : Constant  SampleTime=t
  not_free_wrist3 : Constant  SampleTime=t
  null_space_vetor (fk)1 : Constant  Value=30*[ones(5,1)]  VectorParams1D=off  SampleTime=-1
  null_space_vetor (fk)2 : Constant  Value=50*[ones(4,1)]  VectorParams1D=off  SampleTime=-1
  thumb_convertion : Subsystem
  wrist_convertion : Subsystem
  tau_thumb : Outport
  tau_index : Outport  Port=2
  tau_middle : Outport  Port=3
  tau_ring : Outport  Port=4
  tau_little : Outport  Port=5
  tau_wrist : Outport  Port=6
  wires:
  Slider Gain3/1 -> Mux1/3
  not_free_wrist3/1 -> Slider Gain3/1
  Slider Gain2/1 -> Mux1/2
  not_free_wrist1/1 -> Slider Gain2/1
  Slider Gain1/1 -> Mux1/1
  not_free_wrist2/1 -> Slider Gain1/1
  Mux1/1 -> finger_convertion/1(tau_d)
  .5/1 -> wrist_convertion/1(tau_d)
  .4/1 -> thumb_convertion/1(tau_d)
  finger_convertion/1(fa) -> tau_index/1, Display2/1
  thumb_convertion/1(fa) -> tau_thumb/1
  wrist_convertion/1(fa) -> Mux/1
  Constant/1 -> Mux/2
  Mux/1 -> tau_wrist/1
  .7/1 -> finger_convertion1/1(tau_d)
  finger_convertion1/1(fa) -> tau_middle/1
  .9/1 -> finger_convertion2/1(tau_d)
  finger_convertion2/1(fa) -> tau_ring/1
  .11/1 -> finger_convertion3/1(tau_d)
  finger_convertion3/1(fa) -> tau_little/1
  null_space_vetor (fk)2/1 -> wrist_convertion/2(f0)
  null_space_vetor (fk)1/1 -> finger_convertion3/2(f0), finger_convertion2/2(f0), finger_convertion1/2(f0), finger_convertion/2(f0), thumb_convertion/2(f0)

== system DeathOrGlory/UB Hand system1/Torque filter/First Order Filtering1 ==
  X : Inport
  Fc : Inport  Port=2
  Fs : Inport  Port=3
  reset : Inport  Port=4
  Add2 : Sum  Inputs=++-
  Parameterd calculation1 : Subsystem
  Product1 : Product  Inputs=**  RndMeth=Zero
  Product2 : Product  Inputs=**  RndMeth=Zero
  Product5 : Product  Inputs=**  RndMeth=Zero
  Unit Delay Resettable External IC : simulink_need_slupdate/Unit Delay Resettable External IC  tsamp=-1
      settings: SourceProductName=Simulink  SourceProductBaseCode=SL
  Unit Delay Resettable External IC1 : simulink_need_slupdate/Unit Delay Resettable External IC  tsamp=-1
      settings: SourceProductName=Simulink  SourceProductBaseCode=SL
  reset1 : InportShadow  Port=4
  y : Outport
  wires:
  Fs/1 -> Parameterd calculation1/2(Fs)
  Fc/1 -> Parameterd calculation1/1(Fc)
  Unit Delay Resettable External IC1/1 -> Product2/1
  Product1/1 -> Add2/1
  Product2/1 -> Add2/2
  Product5/1 -> Add2/3
  X/1 -> Unit Delay Resettable External IC1/3, Unit Delay Resettable External IC1/1, Product1/1
  Parameterd calculation1/2(B1) -> Product2/2
  Parameterd calculation1/3(A1) -> Product5/1
  Parameterd calculation1/1(B0) -> Product1/2
  Add2/1 -> Unit Delay Resettable External IC/3, Unit Delay Resettable External IC/1, y/1
  Unit Delay Resettable External IC/1 -> Product5/2
  reset/1 -> Unit Delay Resettable External IC1/2
  reset1/1 -> Unit Delay Resettable External IC/2

== system DeathOrGlory/UB Hand system1/SEND REFERENCES/Joints2Motor/Index_joint2motor ==
  Joint references : Inport
  H_Finger : Inport  Port=2
  Gain2 : Gain  Gain=1/11.5  SampleTime=t
  Matrix Multiply2 : Product  Multiplication=Matrix(*)  SampleTime=t
  mortor references : Outport
  wires:
  Joint references/1 -> Matrix Multiply2/2
  Gain2/1 -> mortor references/1
  Matrix Multiply2/1 -> Gain2/1
  H_Finger/1 -> Matrix Multiply2/1

== system DeathOrGlory/UB Hand system1/SEND REFERENCES/Joints2Motor/Little_joint2motor ==
  Joint references : Inport
  H_Finger : Inport  Port=2
  Gain2 : Gain  Gain=1/11.5  SampleTime=t
  Matrix Multiply2 : Product  Multiplication=Matrix(*)  SampleTime=t
  mortor references : Outport
  wires:
  Matrix Multiply2/1 -> Gain2/1
  Gain2/1 -> mortor references/1
  Joint references/1 -> Matrix Multiply2/2
  H_Finger/1 -> Matrix Multiply2/1

== system DeathOrGlory/UB Hand system1/SEND REFERENCES/Joints2Motor/Middle_joint2motor ==
  Joint references : Inport
  H_Finger : Inport  Port=2
  Gain2 : Gain  Gain=1/11.5  SampleTime=t
  Matrix Multiply2 : Product  Multiplication=Matrix(*)  SampleTime=t
  mortor references : Outport
  wires:
  Matrix Multiply2/1 -> Gain2/1
  Gain2/1 -> mortor references/1
  Joint references/1 -> Matrix Multiply2/2
  H_Finger/1 -> Matrix Multiply2/1

== system DeathOrGlory/UB Hand system1/SEND REFERENCES/Joints2Motor/Ring_joint2motor ==
  Joint references : Inport
  H_Finger : Inport  Port=2
  Gain2 : Gain  Gain=1/11.5  SampleTime=t
  Matrix Multiply2 : Product  Multiplication=Matrix(*)  SampleTime=t
  mortor references : Outport
  wires:
  Joint references/1 -> Matrix Multiply2/2
  Gain2/1 -> mortor references/1
  Matrix Multiply2/1 -> Gain2/1
  H_Finger/1 -> Matrix Multiply2/1

== system DeathOrGlory/UB Hand system1/SEND REFERENCES/Joints2Motor/STORE_INITIAL_OFFSET ==
  control_input : Inport
  initial_position : Inport  Port=2
  Multiport Switch1 : MultiPortSwitch  DataPortOrder=Zero-based contiguous  Inputs=2  DiagnosticForDefault=None
  Unit Delay : UnitDelay  SampleTime=-1
  calibration_offset : Outport
  tag scope: rest_positions=global, trigger_feedback=global
  wires:
  initial_position/1 -> Multiport Switch1/3
  control_input/1 -> [trigger_feedback], Multiport Switch1/1
  Multiport Switch1/1 -> Unit Delay/1
  Unit Delay/1 -> [rest_positions], Multiport Switch1/2, calibration_offset/1

== system DeathOrGlory/UB Hand system1/SEND REFERENCES/Joints2Motor/Thumb_joint2motor ==
  Joint references : Inport
  Gain2 : Gain  Gain=1/11.5  SampleTime=t
  H_FINGER : Constant  Value=[7.34 -11 0;7.34 11 0;0 0 6;-7.34 0 0;0 0 -9.8]  VectorParams1D=off  SampleTime=t
  Matrix Multiply2 : Product  Multiplication=Matrix(*)  SampleTime=t
  mortor references : Outport
  tag scope: H_thumb=global
  wires:
  Matrix Multiply2/1 -> Gain2/1
  H_FINGER/1 -> Matrix Multiply2/1, [H_thumb]
  Gain2/1 -> mortor references/1
  Joint references/1 -> Matrix Multiply2/2

== system DeathOrGlory/UB Hand system1/SEND REFERENCES/Joints2Motor/Wrist_joint2motor ==
  Joint references : Inport
  Gain2 : Gain  Gain=1/11.5  SampleTime=t
  H_FINGER : Constant  Value=[19 0;-19 0;0 12.25;0 -12.25]  VectorParams1D=off  SampleTime=t
  Matrix Multiply2 : Product  Multiplication=Matrix(*)  SampleTime=t
  mortor references : Outport
  tag scope: H_wrist=global
  wires:
  Joint references/1 -> Matrix Multiply2/2
  Gain2/1 -> mortor references/1
  Matrix Multiply2/1 -> Gain2/1
  H_FINGER/1 -> Matrix Multiply2/1, [H_wrist]

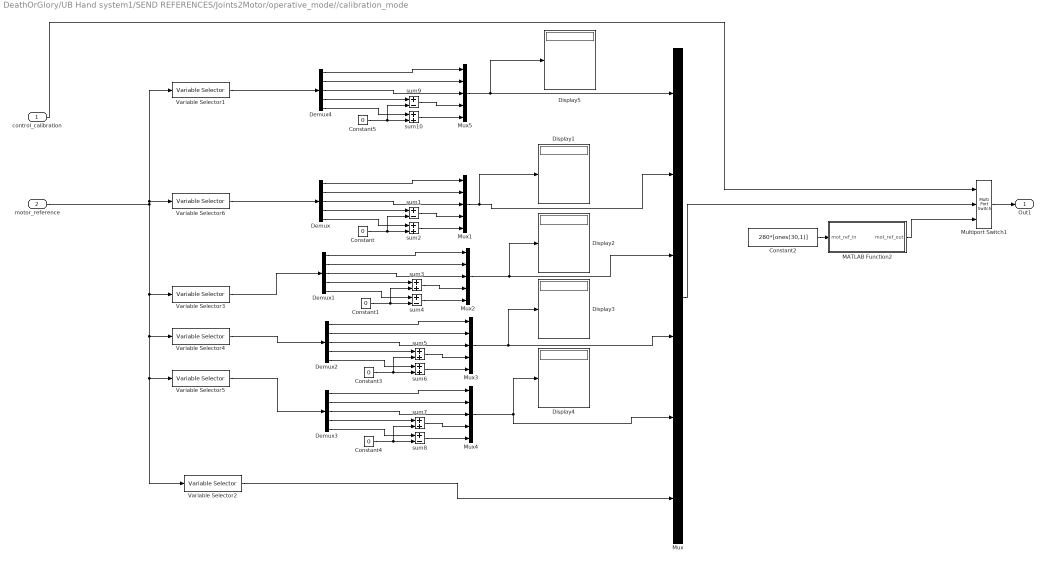
== system DeathOrGlory/UB Hand system1/SEND REFERENCES/Joints2Motor/operative_mode//calibration_mode ==
  control_calibration : Inport
  motor_reference : Inport  Port=2
  Constant{,1,3..5} (5 alike) : Constant  Value=0
  Constant2 : Constant  Value=280*[ones(30,1)]
  Demux{,1..4} (5 alike) : Demux  Outputs=5
  Display{1..5} (5 alike) : Display
  MATLAB Function2 : MATLAB Function  TreatAsAtomicUnit=on
  Multiport Switch1 : MultiPortSwitch  DataPortOrder=Zero-based contiguous  Inputs=2  DiagnosticForDefault=None
  Mux : Mux  Inputs=6
  Mux{1..5} (5 alike) : Mux  Inputs=5
  Variable Selector1 : dspindex/Variable Selector  NumInputs=1  rowsOrCols=Rows  IdxMode=Fixed  Elements=[1:5]  ZerOneIdxMode=One-based  errmode=Clip Index  FillMode=on  FillValues=0
  Variable Selector2 : dspindex/Variable Selector  NumInputs=1  rowsOrCols=Rows  IdxMode=Fixed  Elements=[26:30]  ZerOneIdxMode=One-based  errmode=Clip Index  FillMode=on  FillValues=0
  Variable Selector3 : dspindex/Variable Selector  NumInputs=1  rowsOrCols=Rows  IdxMode=Fixed  Elements=[11:15]  ZerOneIdxMode=One-based  errmode=Clip Index  FillMode=on  FillValues=0
  Variable Selector4 : dspindex/Variable Selector  NumInputs=1  rowsOrCols=Rows  IdxMode=Fixed  Elements=[16:20]  ZerOneIdxMode=One-based  errmode=Clip Index  FillMode=on  FillValues=0
  Variable Selector5 : dspindex/Variable Selector  NumInputs=1  rowsOrCols=Rows  IdxMode=Fixed  Elements=[21:25]  ZerOneIdxMode=One-based  errmode=Clip Index  FillMode=on  FillValues=0
  Variable Selector6 : dspindex/Variable Selector  NumInputs=1  rowsOrCols=Rows  IdxMode=Fixed  Elements=[6:10]  ZerOneIdxMode=One-based  errmode=Clip Index  FillMode=on  FillValues=0
  sum{1,4,8..9} (4 alike) : Sum  Inputs=+-
  sum{2..3,5..7,10} (6 alike) : Sum
  Out1 : Outport
  wires:
  control_calibration/1 -> Multiport Switch1/1
  Constant2/1 -> MATLAB Function2/1(mot_ref_in)
  MATLAB Function2/1(mot_ref_out) -> Multiport Switch1/3
  Multiport Switch1/1 -> Out1/1
  Variable Selector6/1 -> Demux/1
  Mux1/1 -> Display1/1, Mux/2
  Mux/1 -> Multiport Switch1/2
  motor_reference/1 -> Variable Selector1/1, Variable Selector6/1, Variable Selector3/1, Variable Selector4/1, Variable Selector5/1, Variable Selector2/1
  Demux/4 -> sum1/1
  sum1/1 -> Mux1/4
  Demux/5 -> sum2/1
  sum2/1 -> Mux1/5
  Constant/1 -> sum1/2, sum2/2
  Demux/3 -> Mux1/3
  Demux/1 -> Mux1/1
  Demux/2 -> Mux1/2
  Mux2/1 -> Display2/1, Mux/3
  Demux1/4 -> sum3/1
  sum3/1 -> Mux2/4
  Demux1/5 -> sum4/1
  sum4/1 -> Mux2/5
  Constant1/1 -> sum3/2, sum4/2
  Demux1/3 -> Mux2/3
  Demux1/1 -> Mux2/1
  Demux1/2 -> Mux2/2
  Mux3/1 -> Display3/1, Mux/4
  Demux2/4 -> sum5/1
  sum5/1 -> Mux3/4
  Demux2/5 -> sum6/1
  sum6/1 -> Mux3/5
  Constant3/1 -> sum5/2, sum6/2
  Demux2/3 -> Mux3/3
  Demux2/1 -> Mux3/1
  Demux2/2 -> Mux3/2
  Mux4/1 -> Display4/1, Mux/5
  Demux3/4 -> sum7/1
  sum7/1 -> Mux4/4
  Demux3/5 -> sum8/1
  sum8/1 -> Mux4/5
  Constant4/1 -> sum7/2, sum8/2
  Demux3/3 -> Mux4/3
  Demux3/1 -> Mux4/1
  Demux3/2 -> Mux4/2
  Variable Selector2/1 -> Mux/6
  Variable Selector5/1 -> Demux3/1
  Variable Selector4/1 -> Demux2/1
  Variable Selector3/1 -> Demux1/1
  Demux4/4 -> sum9/1
  sum9/1 -> Mux5/4
  Demux4/5 -> sum10/1
  sum10/1 -> Mux5/5
  Constant5/1 -> sum9/2, sum10/2
  Demux4/3 -> Mux5/3
  Demux4/1 -> Mux5/1
  Demux4/2 -> Mux5/2
  Variable Selector1/1 -> Demux4/1
  Mux5/1 -> Display5/1, Mux/1

== system DeathOrGlory/UB Hand system1/SEND REFERENCES/Position_Estimation/Subsystem1 ==
  In1 : Inport
  Add2 : Sum
  Constant21 : Constant  Value=[0 0 0]  SampleTime=-1
  Gain3 : Gain  Gain=11.5
  Matrix Multiply1 : Product  Multiplication=Matrix(*)
  PSEUDO-INV_H_FINGER : Constant  Value=pseudo_inv_h_thumb  VectorParams1D=off  SampleTime=-1
  Out1 : Outport
  wires:
  PSEUDO-INV_H_FINGER/1 -> Matrix Multiply1/1
  Matrix Multiply1/1 -> Gain3/1
  Gain3/1 -> Add2/1
  Constant21/1 -> Add2/2
  Add2/1 -> Out1/1
  In1/1 -> Matrix Multiply1/2

== system DeathOrGlory/UB Hand system1/SEND REFERENCES/Position_Estimation/Subsystem2 ==
  In1 : Inport
  Add2 : Sum
  Constant21 : Constant  Value=[0 0 0]  SampleTime=-1
  Gain3 : Gain  Gain=11.5
  Matrix Multiply1 : Product  Multiplication=Matrix(*)
  PSEUDO-INV_H_FINGER : Constant  Value=pseudo_inv_h_finger  VectorParams1D=off  SampleTime=-1
  Out1 : Outport
  wires:
  In1/1 -> Matrix Multiply1/2
  Add2/1 -> Out1/1
  Constant21/1 -> Add2/2
  Gain3/1 -> Add2/1
  Matrix Multiply1/1 -> Gain3/1
  PSEUDO-INV_H_FINGER/1 -> Matrix Multiply1/1

== system DeathOrGlory/UB Hand system1/SEND REFERENCES/Position_Estimation/Subsystem3 ==
  In1 : Inport
  Add2 : Sum
  Constant21 : Constant  Value=[0 0 0]  SampleTime=-1
  Gain3 : Gain  Gain=11.5
  Matrix Multiply1 : Product  Multiplication=Matrix(*)
  PSEUDO-INV_H_FINGER : Constant  Value=pseudo_inv_h_finger  VectorParams1D=off  SampleTime=-1
  Out1 : Outport
  wires:
  PSEUDO-INV_H_FINGER/1 -> Matrix Multiply1/1
  Matrix Multiply1/1 -> Gain3/1
  Gain3/1 -> Add2/1
  Constant21/1 -> Add2/2
  Add2/1 -> Out1/1
  In1/1 -> Matrix Multiply1/2

== system DeathOrGlory/UB Hand system1/SEND REFERENCES/Position_Estimation/Subsystem4 ==
  In1 : Inport
  Add2 : Sum
  Constant21 : Constant  Value=[0 0 0]  SampleTime=-1
  Gain3 : Gain  Gain=11.5
  Matrix Multiply1 : Product  Multiplication=Matrix(*)
  PSEUDO-INV_H_FINGER : Constant  Value=pseudo_inv_h_finger  VectorParams1D=off  SampleTime=-1
  Out1 : Outport
  wires:
  In1/1 -> Matrix Multiply1/2
  Add2/1 -> Out1/1
  Constant21/1 -> Add2/2
  Gain3/1 -> Add2/1
  Matrix Multiply1/1 -> Gain3/1
  PSEUDO-INV_H_FINGER/1 -> Matrix Multiply1/1

== system DeathOrGlory/UB Hand system1/SEND REFERENCES/Position_Estimation/Subsystem5 ==
  In1 : Inport
  Add2 : Sum
  Constant21 : Constant  Value=[0 0 0]  SampleTime=-1
  Gain3 : Gain  Gain=11.5
  Matrix Multiply1 : Product  Multiplication=Matrix(*)
  PSEUDO-INV_H_FINGER : Constant  Value=pseudo_inv_h_finger  VectorParams1D=off  SampleTime=-1
  Out1 : Outport
  wires:
  PSEUDO-INV_H_FINGER/1 -> Matrix Multiply1/1
  Matrix Multiply1/1 -> Gain3/1
  Gain3/1 -> Add2/1
  Constant21/1 -> Add2/2
  Add2/1 -> Out1/1
  In1/1 -> Matrix Multiply1/2

== system DeathOrGlory/UB Hand system1/SEND REFERENCES/Position_Estimation/Subsystem6 ==
  In1 : Inport
  Add2 : Sum
  Constant21 : Constant  Value=[0 0]  SampleTime=-1
  Gain3 : Gain  Gain=11.5
  Matrix Multiply1 : Product  Multiplication=Matrix(*)
  PSEUDO-INV_H_FINGER : Constant  Value=pseudo_inv_h_wrist  VectorParams1D=off  SampleTime=-1
  Variable Selector : dspindex/Variable Selector  NumInputs=1  rowsOrCols=Rows  IdxMode=Fixed  Elements=[1:4]  ZerOneIdxMode=One-based  errmode=Clip Index  FillMode=on  FillValues=0
  Out1 : Outport
  wires:
  In1/1 -> Variable Selector/1
  Add2/1 -> Out1/1
  Constant21/1 -> Add2/2
  Gain3/1 -> Add2/1
  Matrix Multiply1/1 -> Gain3/1
  PSEUDO-INV_H_FINGER/1 -> Matrix Multiply1/1
  Variable Selector/1 -> Matrix Multiply1/2

== system DeathOrGlory/UB Hand system1/SEND REFERENCES/Subsystem/Triggered Subsystem ==
  Enable : EnablePort
  Level-2 M-file S-Function2 : M-S-Function  FunctionName=dyna_joint_READ  Parameters=[13 14 10 12 11 8 9 7 5 6 2 4 3 27 28 24 26 25 21 23 20 22 19 17 18 15 16 1 30 29] [0 1 0 0 0 0]
  Out2 : Outport
  Out3 : Outport  Port=2
  Out4 : Outport  Port=3
  Out5 : Outport  Port=4
  Out6 : Outport  Port=5
  IsMoving : Outport  Port=6
  wires:
  Level-2 M-file S-Function2/1 -> Out2/1
  Level-2 M-file S-Function2/3 -> Out4/1
  Level-2 M-file S-Function2/4 -> Out5/1
  Level-2 M-file S-Function2/5 -> Out6/1
  Level-2 M-file S-Function2/2 -> Out3/1
  Level-2 M-file S-Function2/6 -> IsMoving/1

== system DeathOrGlory/UB Hand system1/SEND REFERENCES/dyna_send/Subsystem ==
  In1 : Inport
  Add : Sum  Inputs=+-
  Interval Test : simulink/Logic and Bit Operations/Interval Test  IntervalClosedRight=on  uplimit=0.1  IntervalClosedLeft=on  lowlimit=-0.1  OutDataTypeStr=boolean
  Logical Operator : Logic  Operator=NOT  AllPortsSameDT=off  OutDataTypeStr=boolean
  Unit Delay : UnitDelay  InitialCondition=zeros(30,1)  SampleTime=-1
  tag scope: changes_pos=global
  wires:
  Unit Delay/1 -> Add/2
  Add/1 -> Interval Test/1
  Interval Test/1 -> Logical Operator/1
  In1/1 -> Add/1, Unit Delay/1
  Logical Operator/1 -> [changes_pos]

== system DeathOrGlory/UB Hand system1/SEND REFERENCES/dyna_send/Subsystem1 ==
  In1 : Inport
  Add : Sum  Inputs=+-
  Interval Test : simulink/Logic and Bit Operations/Interval Test  IntervalClosedRight=on  uplimit=0.1  IntervalClosedLeft=on  lowlimit=-0.1  OutDataTypeStr=boolean
  Logical Operator : Logic  Operator=NOT  AllPortsSameDT=off  OutDataTypeStr=boolean
  Unit Delay : UnitDelay  InitialCondition=zeros(30,1)  SampleTime=-1
  tag scope: changes_speed=global
  wires:
  Logical Operator/1 -> [changes_speed]
  In1/1 -> Add/1, Unit Delay/1
  Interval Test/1 -> Logical Operator/1
  Add/1 -> Interval Test/1
  Unit Delay/1 -> Add/2

== system DeathOrGlory/UB Hand system1/SEND REFERENCES/dyna_send/Subsystem2 ==
  In1 : Inport
  Add : Sum  Inputs=+-
  Interval Test : simulink/Logic and Bit Operations/Interval Test  IntervalClosedRight=on  uplimit=0.1  IntervalClosedLeft=on  lowlimit=-0.1  OutDataTypeStr=boolean
  Logical Operator : Logic  Operator=NOT  AllPortsSameDT=off  OutDataTypeStr=boolean
  Unit Delay : UnitDelay  InitialCondition=zeros(30,1)  SampleTime=-1
  tag scope: changes_torque=global
  wires:
  Unit Delay/1 -> Add/2
  Add/1 -> Interval Test/1
  Interval Test/1 -> Logical Operator/1
  In1/1 -> Add/1, Unit Delay/1
  Logical Operator/1 -> [changes_torque]

== system DeathOrGlory/UB Hand system1/SEND REFERENCES/dyna_send/Subsystem3 ==
  In1 : Inport
  Add : Sum  Inputs=+-
  Interval Test : simulink/Logic and Bit Operations/Interval Test  IntervalClosedRight=on  uplimit=0.1  IntervalClosedLeft=on  lowlimit=-0.1  OutDataTypeStr=boolean
  Logical Operator : Logic  Operator=NOT  AllPortsSameDT=off  OutDataTypeStr=boolean
  Unit Delay : UnitDelay  InitialCondition=zeros(30,1)  SampleTime=-1
  tag scope: changes_cw_c_m=global
  wires:
  Logical Operator/1 -> [changes_cw_c_m]
  In1/1 -> Add/1, Unit Delay/1
  Interval Test/1 -> Logical Operator/1
  Add/1 -> Interval Test/1
  Unit Delay/1 -> Add/2

== system DeathOrGlory/UB Hand system1/SEND REFERENCES/dyna_send/Subsystem4 ==
  In1 : Inport
  Add : Sum  Inputs=+-
  Interval Test : simulink/Logic and Bit Operations/Interval Test  IntervalClosedRight=on  uplimit=0.1  IntervalClosedLeft=on  lowlimit=-0.1  OutDataTypeStr=boolean
  Logical Operator : Logic  Operator=NOT  AllPortsSameDT=off  OutDataTypeStr=boolean
  Unit Delay : UnitDelay  InitialCondition=zeros(30,1)  SampleTime=-1
  tag scope: changes_cw_c_s=global
  wires:
  Unit Delay/1 -> Add/2
  Add/1 -> Interval Test/1
  Interval Test/1 -> Logical Operator/1
  In1/1 -> Unit Delay/1, Add/1
  Logical Operator/1 -> [changes_cw_c_s]

== system DeathOrGlory/UB Hand system1/SEND REFERENCES/dyna_send/Subsystem5 ==
  In1 : Inport
  Add : Sum  Inputs=+-
  Interval Test : simulink/Logic and Bit Operations/Interval Test  IntervalClosedRight=on  uplimit=0.1  IntervalClosedLeft=on  lowlimit=-0.1  OutDataTypeStr=boolean
  Logical Operator : Logic  Operator=NOT  AllPortsSameDT=off  OutDataTypeStr=boolean
  Unit Delay : UnitDelay  InitialCondition=zeros(30,1)  SampleTime=-1
  tag scope: changes_ccw_c_m=global
  wires:
  Unit Delay/1 -> Add/2
  Add/1 -> Interval Test/1
  Interval Test/1 -> Logical Operator/1
  In1/1 -> Unit Delay/1, Add/1
  Logical Operator/1 -> [changes_ccw_c_m]

== system DeathOrGlory/UB Hand system1/SEND REFERENCES/dyna_send/Subsystem6 ==
  In1 : Inport
  Add : Sum  Inputs=+-
  Interval Test : simulink/Logic and Bit Operations/Interval Test  IntervalClosedRight=on  uplimit=0.1  IntervalClosedLeft=on  lowlimit=-0.1  OutDataTypeStr=boolean
  Logical Operator : Logic  Operator=NOT  AllPortsSameDT=off  OutDataTypeStr=boolean
  Unit Delay : UnitDelay  InitialCondition=zeros(30,1)  SampleTime=-1
  tag scope: changes_ccw_c_s=global
  wires:
  Logical Operator/1 -> [changes_ccw_c_s]
  In1/1 -> Add/1, Unit Delay/1
  Interval Test/1 -> Logical Operator/1
  Add/1 -> Interval Test/1
  Unit Delay/1 -> Add/2
